simulink model "PDInverseDyn"  (R2020b)
settings: Solver=VariableStepAuto  StartTime=0.0  StopTime=5  RelTol=1e-3
values from neighbouring files (symbols this model uses):
  Kd = diag([200 40 15])    [params.m]
  Kp = diag([600 380 250])    [params.m]
libraries: robotcorelib x1
settings Model: Creator=andre  LastModifiedBy=filippo

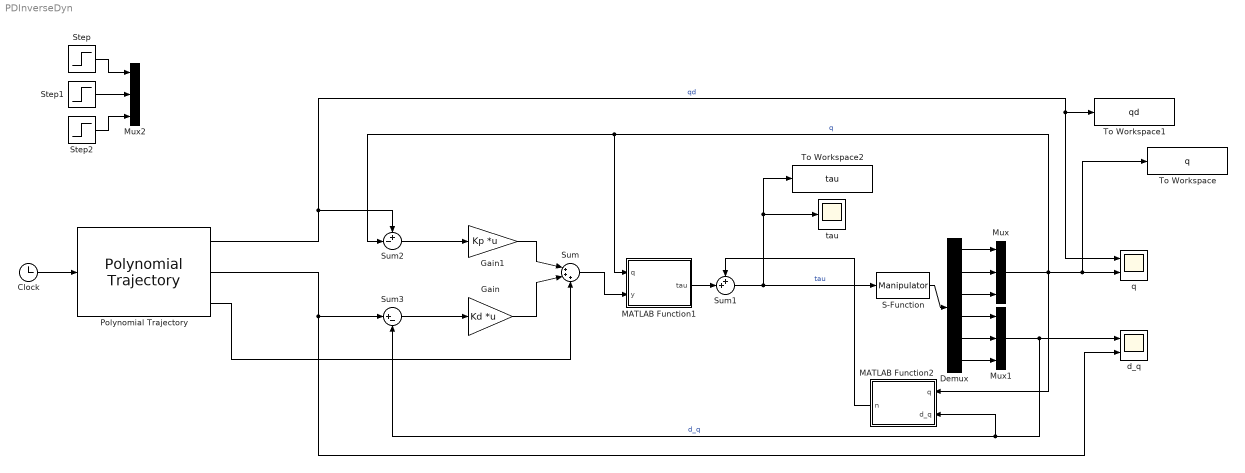
== system PDInverseDyn ==
  Clock : Clock
  Demux : Demux  Outputs=6
  Gain : Gain  Gain=Kd  Multiplication=Matrix(K*u)
  Gain1 : Gain  Gain=Kp  Multiplication=Matrix(K*u)
  MATLAB Function1 : MATLAB Function  TreatAsAtomicUnit=on
  MATLAB Function2 : MATLAB Function  TreatAsAtomicUnit=on
  Mux : Mux  Inputs=3
  Mux1 : Mux  Inputs=3
  Mux2 : Mux  Inputs=3
  Polynomial Trajectory : robotcorelib/Polynomial Trajectory  WaypointSource=Internal  Waypoints=[ 0, 0.3, 0.1; 0, -0.1, -0.05; 0, 0.1, 0]  TimePoints=[ 0, 3, 5 ]  TimeInterval=[ 1, 4 ]  Method=Quintic Polynomial  ParameterSource=Internal  VelocityBoundaryCondition=zeros( 3, 3 )  AccelerationBoundaryCondition=zeros( 3, 3 )  SimulateUsing=Interpreted execution
  S-Function : S-Function  FunctionName=Manipulator  Parameters=param  SFunctionDeploymentMode=off  EnableBusSupport=off
  Step : Step  After=0.1  SampleTime=0
  Step1 : Step  After=0.1  SampleTime=0
  Step2 : Step  After=0.1  SampleTime=0
  Sum : Sum  Inputs=|+++
  Sum1 : Sum  Inputs=++|
  Sum2 : Sum  Inputs=+-|
  Sum3 : Sum  Inputs=|+-
  To Workspace : ToWorkspace  VariableName=q  SaveFormat=Timeseries  SampleTime=-1
  To Workspace1 : ToWorkspace  VariableName=qd  SaveFormat=Timeseries  SampleTime=-1
  To Workspace2 : ToWorkspace  VariableName=tau  SaveFormat=Timeseries  SampleTime=-1
  d_q : Scope  NumInputPorts=2
  q : Scope  NumInputPorts=2
  tau : Scope
  wires:
  Gain1/1 -> Sum/1
  S-Function/1 -> Demux/1
  Demux/3 -> Mux/3
  Demux/2 -> Mux/2
  Demux/1 -> Mux/1
  Demux/4 -> Mux1/1
  Demux/5 -> Mux1/2
  Demux/6 -> Mux1/3
  Mux/1 -> MATLAB Function2/1(q), Sum2/2, MATLAB Function1/1(q), To Workspace/1, q/2  "q"
  Sum1/1 -> To Workspace2/1, tau/1, S-Function/1  "tau"
  Gain/1 -> Sum/2
  Mux1/1 -> Sum3/2, MATLAB Function2/2(d_q), d_q/1  "d_q"
  MATLAB Function2/1(n) -> Sum1/1
  MATLAB Function1/1(tau) -> Sum1/2
  Sum/1 -> MATLAB Function1/2(y)
  Sum2/1 -> Gain1/1
  Sum3/1 -> Gain/1
  Polynomial Trajectory/1 -> q/1, To Workspace1/1, Sum2/1  "qd"
  Polynomial Trajectory/2 -> d_q/2, Sum3/1
  Clock/1 -> Polynomial Trajectory/1
  Polynomial Trajectory/3 -> Sum/3
  Step/1 -> Mux2/1
  Step1/1 -> Mux2/2
  Step2/1 -> Mux2/3

== matlab function PDInverseDyn/MATLAB Function1 ==
  data: q input; y input; tau output; param parameter
function tau = B(q,y,param)

    % Change the parameter of the masses in the achitecture
%     param.m1 = param.m1*2;
%     param.m3 = param.m3*2;
    
    B_matrix = B_Lagrangian(q, param);
    tau =  B_matrix * y;
end

== matlab function PDInverseDyn/MATLAB Function2 ==
  data: q input; n output; d_q input; param parameter
function n = n(q,d_q,param)
    % Compute C and G used in the model of n(q,d_q)
    
    % Change the parameter of the masses in the achitecture
%     param.m1 = param.m1*2;
%     param.m3 = param.m3*2;
    
    C = double(C_Lagrangian(q, d_q, param));
    G = double(G_Lagrangian(q, param));
    Fsv = param.Fsv;

    n = C * d_q + G + Fsv * d_q;
end
